simulink model "act1"  (R2021a)
settings: Solver=ode1  StartTime=0.0  StopTime=10.0  FixedStep=0.1  RelTol=1e-3
values from neighbouring files (symbols this model uses):
  a1 = 2    [exp1.m]
  a2 = 1    [exp1.m]
settings Model: Creator=zeta  LastModifiedBy=Agus

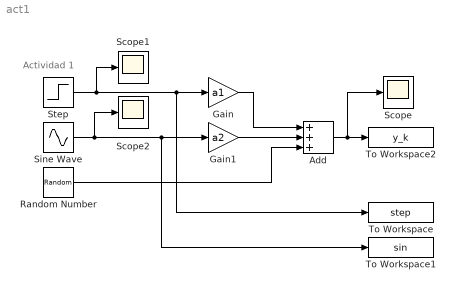
== system act1 ==
  note: Actividad 1
  Add : Sum  Inputs=+++
  Gain : Gain  Gain=a1
  Gain1 : Gain  Gain=a2
  Random Number : RandomNumber  Variance=0.1  Seed=round(rand()*100)  SampleTime=0.1
  Scope : Scope
  Scope1 : Scope
  Scope2 : Scope
  Sine Wave : Sin  Frequency=10  SampleTime=0
  Step : Step  SampleTime=0
  To Workspace : ToWorkspace  VariableName=step  SampleTime=0.5
  To Workspace1 : ToWorkspace  VariableName=sin  SampleTime=0.5
  To Workspace2 : ToWorkspace  VariableName=y_k  SampleTime=0.5
  wires:
  Step/1 -> Scope1/1, To Workspace/1, Gain/1
  Sine Wave/1 -> Scope2/1, Gain1/1, To Workspace1/1
  Gain1/1 -> Add/2
  Gain/1 -> Add/1
  Add/1 -> Scope/1, To Workspace2/1
  Random Number/1 -> Add/3
